simulink model "QCar2_Manual_Drive"  (R2023a)
settings: Solver=ode2  StartTime=0.0  StopTime=inf  FixedStep=1/100  RelTol=1e-3  EnableMultiTasking=on
undefined symbols (not defined in the file): HIL, Host, qc_get_step_size
libraries: quarc_library x15, simulink x13
settings Model: SimulationMode=external  ExtModeTrigDuration=10000  Creator=mbohra  LastModifiedBy=ZinanCen
settings SolverCC: AlgebraicLoopSolver=TrustRegion  PositivePriorityOrder=on
settings DataIOCC: SaveOutput=off  SignalLogging=off  DSMLogging=off  SaveTime=off  ReturnWorkspaceOutputs=off
settings DebuggingCC: UnconnectedInputMsg=warning  UnconnectedOutputMsg=warning  UnconnectedLineMsg=warning  ArithmeticOperatorsInVariantConditions=warning
settings ModelReferenceCC: EnableRefExpFcnMdlSchedulingChecks=on
settings SFSimCC: CustomCodeUndefinedFunction=UseInterfaceOnly
settings RTWCC: Toolchain=QUARC win64 | nmake (64-bit Windows)  BuildConfiguration=Faster Runs

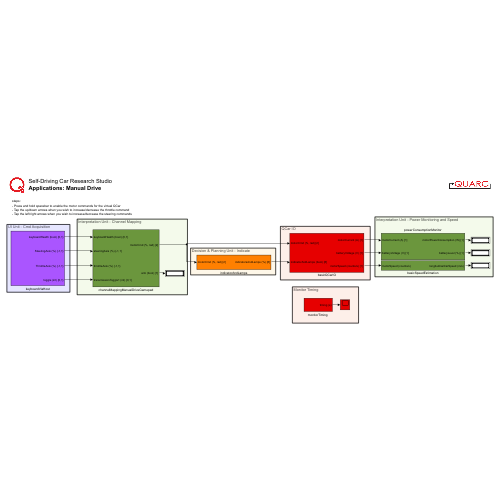
[thumbnail: Simulink's stored preview of the top-level diagram]
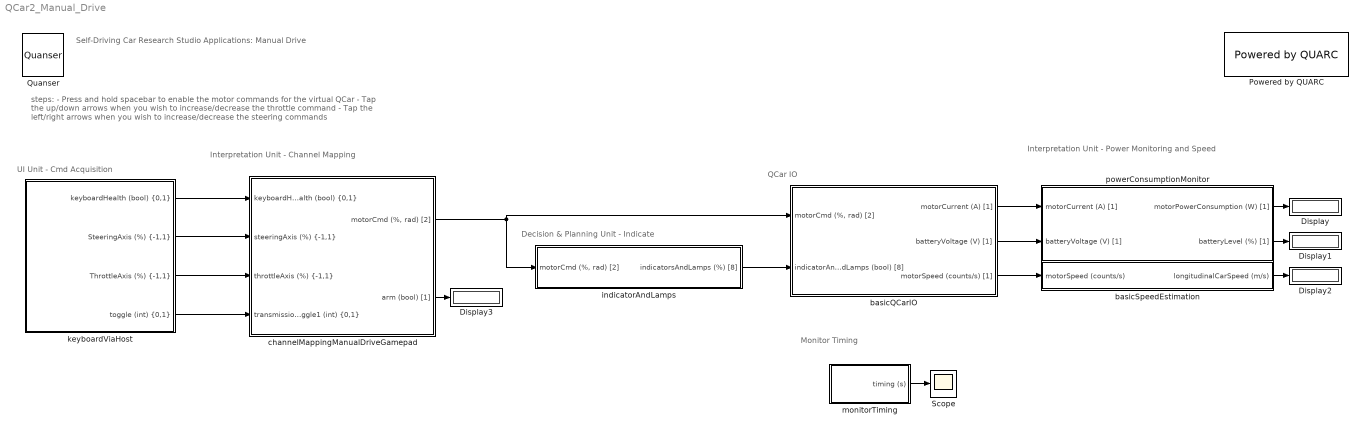
== system QCar2_Manual_Drive ==
  note: steps:
      | - Press and hold spacebar to enable the motor commands for the virtual QCar
      | - Tap the up/down arrows when you wish to increase/decrease the throttle command
      | - Tap the left/right arrows when you wish to increase/decrease the steering commands
  note: Monitor Timing
  note: Decision & Planning Unit - Indicate
  note: Interpretation Unit - Channel Mapping
  note: Interpretation Unit - Power Monitoring and Speed
  note: QCar IO
  note: UI Unit - Cmd Acquisition
  note: Self-Driving Car Research Studio
      | Applications: Manual Drive
  Display{,1..3} (4 alike) : Display
      Display settings: Decimation=0.5/qc_get_step_size
      Display1 settings: Decimation=0.5/qc_get_step_size
      Display2 settings: Decimation=0.5/qc_get_step_size
      Display3 settings: Decimation=0.1/qc_get_step_size
  Powered by QUARC : quarc_library/Logos/Powered by QUARC
  Quanser : quarc_library/Logos/Quanser
  Scope : Scope
  basicQCarIO : Subsystem
  basicSpeedEstimation : Subsystem
  channelMappingManualDriveGamepad : Subsystem
  indicatorAndLamps : Subsystem
  keyboardViaHost : Subsystem
  "monitorTiming " : Subsystem
  powerConsumptionMonitor : Subsystem
  wires:
  indicatorAndLamps/1(indicatorsAndLamps (%) [8]) -> basicQCarIO/2(indicatorAndLamps (bool) [8])
  keyboardViaHost/1("keyboardHealth (bool) {0,1}") -> channelMappingManualDriveGamepad/1("keyboardHealth (bool) {0,1}")
  channelMappingManualDriveGamepad/2(arm (bool) [1]) -> Display3/1
  basicQCarIO/3(motorSpeed (counts/s) [1]) -> basicSpeedEstimation/1(motorSpeed (counts/s))
  basicQCarIO/1(motorCurrent (A) [1]) -> powerConsumptionMonitor/1(motorCurrent (A) [1])
  basicQCarIO/2(batteryVoltage (V) [1]) -> powerConsumptionMonitor/2(batteryVoltage (V) [1])
  basicSpeedEstimation/1(longitudinalCarSpeed (m/s)) -> Display2/1
  powerConsumptionMonitor/2(batteryLevel (%) [1]) -> Display1/1
  powerConsumptionMonitor/1(motorPowerConsumption (W) [1]) -> Display/1
  "monitorTiming "/1(timing (s)) -> Scope/1
  channelMappingManualDriveGamepad/1("motorCmd (%, rad) [2]") -> basicQCarIO/1("motorCmd (%, rad) [2]"), indicatorAndLamps/1("motorCmd (%, rad) [2]")
  keyboardViaHost/3("ThrottleAxis (%) {-1,1}") -> channelMappingManualDriveGamepad/3("throttleAxis (%) {-1,1}")
  keyboardViaHost/2("SteeringAxis (%) {-1,1}") -> channelMappingManualDriveGamepad/2("steeringAxis (%) {-1,1}")
  keyboardViaHost/4("toggle (int) {0,1}") -> channelMappingManualDriveGamepad/4("transmissionToggle1 (int) {0,1}")

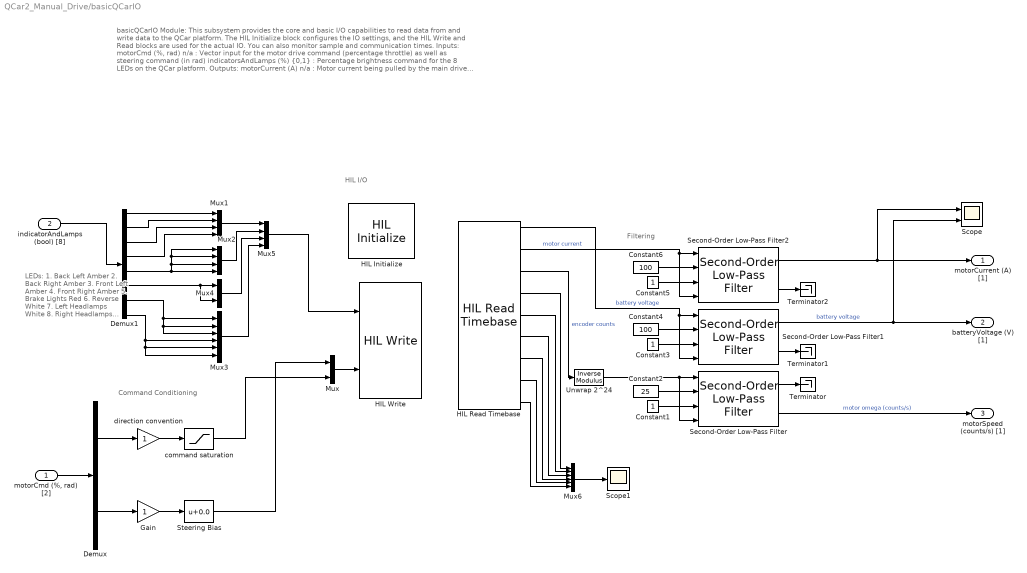
== system QCar2_Manual_Drive/basicQCarIO ==
  note: Filtering
  note: basicQCarIO Module:
      |
      | This subsystem provides the core and basic I/O capabilities to read data from and write data to the QCar platform. The HIL Initialize block configures the IO settings, and the HIL Write and Read blocks are used for the actual IO. You can also monitor sample and communication times.
      |
      | Inputs:
      | motorCmd (%, rad) n/a : Vector input for the motor drive command (percentage throttle) as well as steering command (in rad)
      | indicatorsAndLamps (%) {0,1} : Percentage brightness command for the 8 LEDs on the QCar platform.
      |
      | Outputs:
      | motorCurrent (A) n/a : Motor current being pulled by the main drive motor
      | batteryVoltage (V) {0, 12.6} : Current battery voltage reading
      | motorSpeed (counts/s) n/a : Drive motor speed measured using an encoder (do not confuse with wheel speed as this measurement is at the drive shaft)
  note: HIL I/O
  note: Command Conditioning
  note: LEDs:
      | 1. Back Left Amber
      | 2. Back Right Amber
      | 3. Front Left Amber
      | 4. Front Right Amber
      | 5. Brake Lights Red
      | 6. Reverse White
      | 7. Left Headlamps White
      | 8. Right Headlamps White
  "motorCmd (%, rad) [2]" : Inport
  indicatorAndLamps (bool) [8] : Inport  Port=2
  Constant1 : Constant
  Constant2 : Constant  Value=25
  Constant3 : Constant
  Constant4 : Constant  Value=100
  Constant5 : Constant
  Constant6 : Constant  Value=100
  Demux : Demux  Outputs=2
  Demux1 : Demux  Outputs=8
  Gain : Gain
  HIL Initialize : quarc_library/Data Acquisition/Generic/Configuration/HIL Initialize  object_name=HIL-1  board_type=qcar2  board_number=0@tcpip://localhost:18960  board_options=gyro_fs=250;gyro_rate=500;gyro_bw=125;gyro_ord=3;accel_fs=16;accel_rate=1000;accel_bw=250;accel_ord=3;temp_bw=4000;enc0_dir=0;enc1_dir=0;enc2_dir=0;steer_bias=0.05;  exclusive=off  active=on  hardware_clocks=[]  clock_modes=[]  initial_clock_frequencies=[]  set_clock_params_at_start=off  set_clock_params_at_switch_in=off  set_clock_frequencies_at_start=off  set_clock_frequencies_at_switch_in=off  analog_input_channels=[0:4]  analog_input_configurations=[]  analog_input_maximums=[3.3]  analog_input_minimums=[0]  set_analog_input_params_at_start=off  set_analog_input_params_at_switch_in=off  analog_output_channels=[]  analog_output_maximums=[]  analog_output_minimums=[]  initial_analog_outputs=[]  final_analog_outputs=[]  watchdog_analog_outputs=[]  set_analog_output_params_at_start=off  set_analog_output_params_at_switch_in=off  set_analog_outputs_at_start=off  set_analog_outputs_at_switch_in=off  set_analog_outputs_at_terminate=off  set_analog_outputs_at_switch_out=off  set_analog_outputs_on_watchdog=off  digital_input_channels=[0:14]  digital_output_channels=[11:26]  digital_output_configuration=[]  initial_digital_outputs=[0]  final_digital_outputs=[0]  watchdog_digital_outputs=[0]  set_digital_output_params_at_start=off  set_digital_output_params_at_switch_in=off  set_digital_outputs_at_start=on  set_digital_outputs_at_switch_in=off  set_digital_outputs_at_terminate=on  set_digital_outputs_at_switch_out=off  set_digital_outputs_on_watchdog=off  encoder_channels=[0:2]  quadrature=[4]  encoder_filter_frequency=100e6/1  initial_encoder_counts=[0]  set_encoder_params_at_start=on  set_encoder_params_at_switch_in=off  set_encoder_counts_at_start=on  set_encoder_counts_at_switch_in=off  pwm_channels=[0:1]  pwm_modes=[0]  pwm_frequency=180e6/4096  pwm_configuration=[0]  pwm_alignment=[0]  pwm_polarity=[1]  pwm_leading_deadband=[]  pwm_trailing_deadband=[]  initial_pwm_outputs=[0]  final_pwm_outputs=[0]  watchdog_pwm_outputs=[0]  set_pwm_params_at_start=on  set_pwm_params_at_switch_in=off  set_pwm_outputs_at_start=on  set_pwm_outputs_at_switch_in=off  set_pwm_outputs_at_terminate=on  set_pwm_outputs_at_switch_out=off  set_pwm_outputs_on_watchdog=off  other_output_channels=[1000 11000]  initial_other_outputs=[0]  final_other_outputs=[0]  watchdog_other_outputs=[0]  set_other_outputs_at_start=on  set_other_outputs_at_switch_in=off  set_other_outputs_at_terminate=on  set_other_outputs_at_switch_out=off  set_other_outputs_on_watchdog=off
  HIL Read Timebase : quarc_library/Data Acquisition/Generic/Timebases/HIL Read Timebase  object_name=HIL-1  clock=0  analog_channels=[2 4]  encoder_channels=[0]  digital_channels=[]  other_channels=[3000:3002 4000:4002]  active=on  vector_output=off  data_type_mode=Inherit via back propagation  encoder_data_type=double  digital_data_type=boolean  overflow_mode=Synchronize (for simulated cards only)  samples_in_buffer=max(ceil(1/qc_get_step_size), 1)*0+1
  HIL Write : quarc_library/Data Acquisition/Generic/Immediate I//O/HIL Write  object_name=HIL-1  analog_channels=[]  pwm_channels=[]  digital_channels=[17:18 25:26 11:16 19:24]  other_channels=[1000 11000]  sample_time=qc_get_step_size  active=on  vector_input=on
  Mux : Mux  Inputs=2
  Mux1 : Mux
  Mux2 : Mux
  Mux3 : Mux  Inputs=6
  Mux4 : Mux  Inputs=2
  Mux5 : Mux
  Mux6 : Mux  Inputs=6
  Scope : Scope  NumInputPorts=2
  Scope1 : Scope
  Second-Order Low-Pass Filter : quarc_library/Continuous/Second-Order Low-Pass Filter  params_source=External (input ports)  input_width=1  input_zeta=1  input_init=0
  Second-Order Low-Pass Filter1 : quarc_library/Continuous/Second-Order Low-Pass Filter  params_source=External (input ports)  input_width=1  input_zeta=1  input_init=0
  Second-Order Low-Pass Filter2 : quarc_library/Continuous/Second-Order Low-Pass Filter  params_source=External (input ports)  input_width=1  input_zeta=1  input_init=0
  Steering Bias : Bias  Bias=0.0  SaturateOnIntegerOverflow=off
  Terminator : Terminator
  Terminator1 : Terminator
  Terminator2 : Terminator
  Unwrap 2^24 : quarc_library/Discontinuities/Inverse Modulus  modulus=16777215  output_derivative=off  output_revolutions=off  max_x=Inf  min_x=-Inf
  command saturation : Saturate  UpperLimit=0.20  LowerLimit=-0.20
  direction convention : Gain
  motorCurrent (A) [1] : Outport  VectorParamsAs1DForOutWhenUnconnected=off
  batteryVoltage (V) [1] : Outport  Port=2  VectorParamsAs1DForOutWhenUnconnected=off
  motorSpeed (counts/s) [1] : Outport  Port=3  VectorParamsAs1DForOutWhenUnconnected=off
  wires:
  Second-Order Low-Pass Filter2/1 -> Scope/1, motorCurrent (A) [1]/1
  Constant2/1 -> Second-Order Low-Pass Filter/2
  Unwrap 2^24/1 -> Second-Order Low-Pass Filter/1, Second-Order Low-Pass Filter/4
  Second-Order Low-Pass Filter/1 -> Terminator/1
  Constant3/1 -> Second-Order Low-Pass Filter1/3
  Second-Order Low-Pass Filter1/1 -> Scope/2, batteryVoltage (V) [1]/1  "battery voltage"
  Constant5/1 -> Second-Order Low-Pass Filter2/3
  Second-Order Low-Pass Filter1/2 -> Terminator1/1
  HIL Read Timebase/1 -> Second-Order Low-Pass Filter1/4, Second-Order Low-Pass Filter1/1  "battery voltage"
  Constant6/1 -> Second-Order Low-Pass Filter2/2
  Second-Order Low-Pass Filter/2 -> motorSpeed (counts/s) [1]/1  "motor omega (counts/s)"
  Second-Order Low-Pass Filter2/2 -> Terminator2/1
  Constant4/1 -> Second-Order Low-Pass Filter1/2
  Constant1/1 -> Second-Order Low-Pass Filter/3
  HIL Read Timebase/3 -> Unwrap 2^24/1  "encoder counts"
  HIL Read Timebase/2 -> Second-Order Low-Pass Filter2/1, Second-Order Low-Pass Filter2/4  "motor current"
  Mux5/1 -> HIL Write/1
  "motorCmd (%, rad) [2]"/1 -> Demux/1
  Mux3/1 -> Mux5/4
  Demux1/4 -> Mux1/4
  Demux1/3 -> Mux1/3
  Demux1/6 -> Mux4/2, Mux4/1
  Steering Bias/1 -> Mux/1
  Demux1/8 -> Mux3/5, Mux3/6, Mux3/4
  Mux1/1 -> Mux5/1
  Demux1/7 -> Mux3/2, Mux3/3, Mux3/1
  Demux/1 -> direction convention/1
  Demux1/5 -> Mux2/4, Mux2/3, Mux2/2, Mux2/1
  Mux2/1 -> Mux5/2
  Mux/1 -> HIL Write/2
  indicatorAndLamps (bool) [8]/1 -> Demux1/1
  Demux/2 -> Gain/1
  Mux4/1 -> Mux5/3
  command saturation/1 -> Mux/2
  Demux1/2 -> Mux1/2
  direction convention/1 -> command saturation/1
  Gain/1 -> Steering Bias/1
  Demux1/1 -> Mux1/1
  Mux6/1 -> Scope1/1
  HIL Read Timebase/9 -> Mux6/6
  HIL Read Timebase/7 -> Mux6/4
  HIL Read Timebase/5 -> Mux6/2
  HIL Read Timebase/8 -> Mux6/5
  HIL Read Timebase/6 -> Mux6/3
  HIL Read Timebase/4 -> Mux6/1

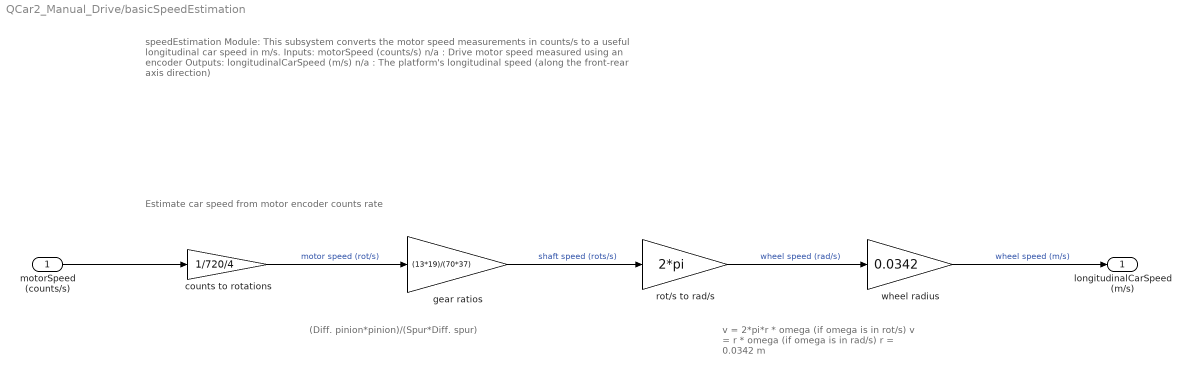
== system QCar2_Manual_Drive/basicSpeedEstimation ==
  note: speedEstimation Module:
      |
      | This subsystem converts the motor speed measurements in counts/s to a useful longitudinal car speed in m/s.
      |
      | Inputs:
      | motorSpeed (counts/s) n/a : Drive motor speed measured using an encoder
      |
      | Outputs:
      | longitudinalCarSpeed (m/s) n/a : The platform's longitudinal speed (along the front-rear axis direction)
  note: (Diff. pinion*pinion)/(Spur*Diff. spur)
  note: v = 2*pi*r * omega (if omega is in rot/s)
      | v = r * omega (if omega is in rad/s)
      | r = 0.0342 m
  note: Estimate car speed from motor encoder counts rate
  motorSpeed (counts/s) : Inport
  counts to rotations : Gain  Gain=1/720/4
  gear ratios : Gain  Gain=(13*19)/(70*37)
  rot/s to rad/s : Gain  Gain=2*pi
  wheel radius : Gain  Gain=0.0342
  longitudinalCarSpeed (m/s) : Outport  VectorParamsAs1DForOutWhenUnconnected=off
  wires:
  gear ratios/1 -> rot/s to rad/s/1  "shaft speed (rots/s)"
  wheel radius/1 -> longitudinalCarSpeed (m/s)/1  "wheel speed (m/s)"
  counts to rotations/1 -> gear ratios/1  "motor speed (rot/s)"
  rot/s to rad/s/1 -> wheel radius/1  "wheel speed (rad/s)"
  motorSpeed (counts/s)/1 -> counts to rotations/1

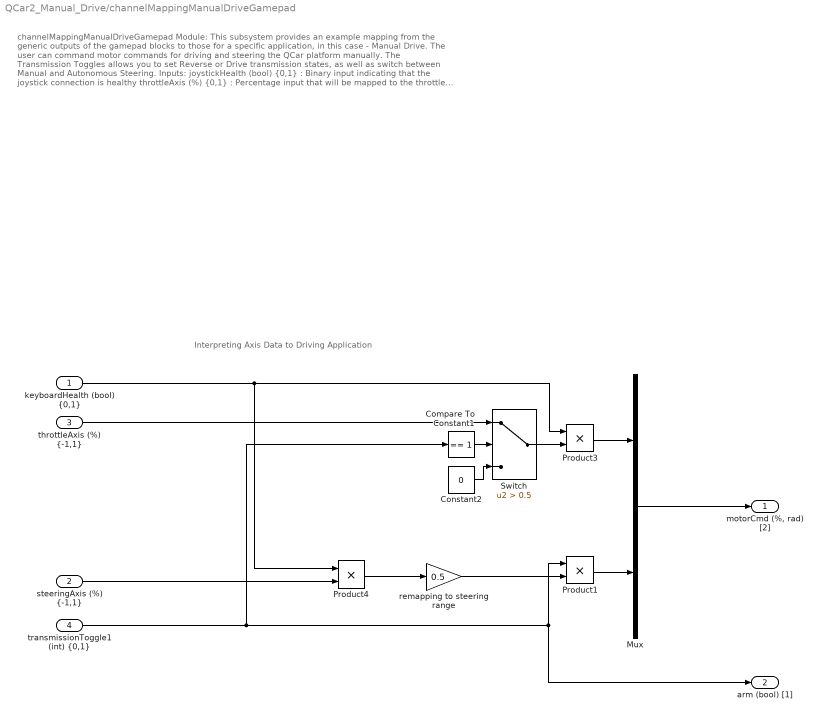
== system QCar2_Manual_Drive/channelMappingManualDriveGamepad ==
  note: channelMappingManualDriveGamepad Module:
      |
      | This subsystem provides an example mapping from the generic outputs of the gamepad blocks to those for a specific application, in this case - Manual Drive. The user can command motor commands for driving and steering the QCar platform manually. The Transmission Toggles allows you to set Reverse or Drive transmission states, as well as switch between Manual and Autonomous Steering.
      |
      | Inputs:
      | joystickHealth (bool) {0,1} : Binary input indicating that the joystick connection is healthy
      | throttleAxis (%) {0,1} : Percentage input that will be mapped to the throttle command
      | steeringAxis (%) {-1,1} : Signed percentage input that will be mapped to steering
      | transmissionToggle1 (int) {0,1} : 2-state input that will decide the Park/Engage State
      | transmissionToggle2 (int) {0, 1} : 2-state input that will decide the Reverse/Drive State
      |
      | Outputs:
      | motorCmd (%, rad) n/a : Vector output for the motor drive command (percentage throttle) as well as steering command (in rad)
      | arm (bool) {0,1} : Binary output indicating status (armed or disarmed)
      |
      | Usage:
      | 1. When the Transmission Toggle 1 input
      | a. reads 1, the Arm output will be high (1), which is the Armed state.
      | b. reads 0, the Arm output will be low (0), which is the Disarmed state.
      | 2. In addition, the Transmission Toggle 2 input
      | a. reading 0 is the Drive state, and the Motor Cmd for the throttle will range from 0 to 100%, spinning the wheels forwards.
      | b. reading 1 is the Reverse state, and the Motor Cmd for the throttle will range from 0 to -100%, spinning the wheels backwards.
  note: Interpreting Axis Data to Driving Application
  "keyboardHealth (bool) {0,1}" : Inport
  "steeringAxis (%) {-1,1}" : Inport  Port=2
  "throttleAxis (%) {-1,1}" : Inport  Port=3
  "transmissionToggle1 (int) {0,1}" : Inport  Port=4
  " remapping to steering range " : Gain  Gain=0.5
  Compare To Constant1 : simulink/Logic and Bit Operations/Compare To Constant  relop===  const=1  OutDataTypeStr=boolean
  Constant2 : Constant  Value=0
  Mux : Mux  Inputs=2
  Product1 : Product
  Product3 : Product
  Product4 : Product
  Switch : Switch  Criteria=u2 > Threshold  Threshold=0.5  SaturateOnIntegerOverflow=off  InputSameDT=off
  "motorCmd (%, rad) [2]" : Outport  VectorParamsAs1DForOutWhenUnconnected=off
  arm (bool) [1] : Outport  Port=2  VectorParamsAs1DForOutWhenUnconnected=off
  wires:
  Switch/1 -> Product3/2
  Product1/1 -> Mux/2
  Compare To Constant1/1 -> Switch/2
  "steeringAxis (%) {-1,1}"/1 -> Product4/2
  "keyboardHealth (bool) {0,1}"/1 -> Product4/1, Product3/1
  "transmissionToggle1 (int) {0,1}"/1 -> Compare To Constant1/1, Product1/1, arm (bool) [1]/1
  Product3/1 -> Mux/1
  " remapping to steering range "/1 -> Product1/2
  Product4/1 -> " remapping to steering range "/1
  Mux/1 -> "motorCmd (%, rad) [2]"/1
  "throttleAxis (%) {-1,1}"/1 -> Switch/1
  Constant2/1 -> Switch/3

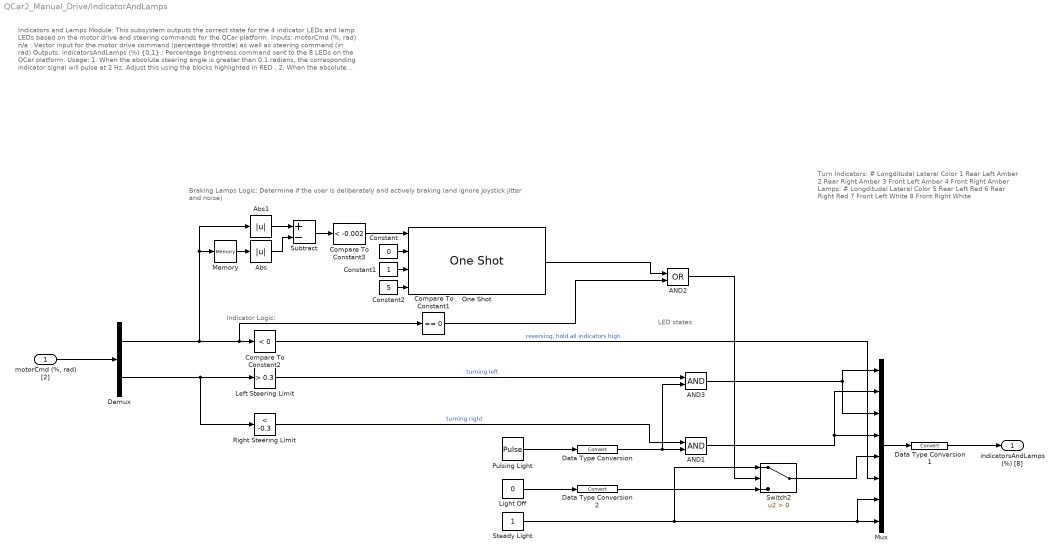
== system QCar2_Manual_Drive/indicatorAndLamps ==
  note: Indicators and Lamps Module:
      |
      | This subsystem outputs the correct state for the 4 indicator LEDs and lamp LEDs based on the motor drive and steering commands for the QCar platform.
      |
      | Inputs:
      | motorCmd (%, rad) n/a : Vector input for the motor drive command (percentage throttle) as well as steering command (in rad)
      |
      | Outputs:
      | indicatorsAndLamps (%) {0,1} : Percentage brightness command sent to the 8 LEDs on the QCar platform.
      |
      | Usage:
      | 1. When the absolute steering angle is greater than 0.1 radians, the corresponding indicator signal will pulse at 2 Hz. Adjust this using the blocks highlighted in RED .
      | 2. When the absolute motor drive command approaches 0, the brake lamps will receive 100% brightness command, and 0% brightness otherwise. Adjust this using the blocks highlighted in GREEN .
  note: Braking Lamps Logic:
      | Determine if the user is deliberately and actively braking (and ignore joystick jitter and noise)
  note: LED states
  note: Turn Indicators:
      | # Longditudal Lateral Color
      | 1 Rear Left Amber
      | 2 Rear Right Amber
      | 3 Front Left Amber
      | 4 Front Right Amber
      |
      | Lamps:
      | # Longditudal Lateral Color
      | 5 Rear Left Red
      | 6 Rear Right Red
      | 7 Front Left White
      | 8 Front Right White
  note: Indicator Logic:
  "motorCmd (%, rad) [2]" : Inport
  AND1 : Logic  IconShape=distinctive  AllPortsSameDT=off  OutDataTypeStr=boolean
  AND2 : Logic  Operator=OR  IconShape=distinctive  AllPortsSameDT=off  OutDataTypeStr=boolean
  AND3 : Logic  IconShape=distinctive  AllPortsSameDT=off  OutDataTypeStr=boolean
  Abs : Abs  SaturateOnIntegerOverflow=off
  Abs1 : Abs  SaturateOnIntegerOverflow=off
  Compare To Constant1 : simulink/Logic and Bit Operations/Compare To Constant  relop===  const=0  OutDataTypeStr=uint8
  Compare To Constant2 : simulink/Logic and Bit Operations/Compare To Constant  relop=<  const=0  OutDataTypeStr=boolean
  Compare To Constant3 : simulink/Logic and Bit Operations/Compare To Constant  relop=<  const=-0.002  OutDataTypeStr=boolean
  Constant : Constant  Value=0
  Constant1 : Constant
  Constant2 : Constant  Value=5
  Data Type Conversion : DataTypeConversion  SaturateOnIntegerOverflow=off  RndMeth=Floor
  Data Type Conversion1 : DataTypeConversion  SaturateOnIntegerOverflow=off  RndMeth=Floor
  Data Type Conversion2 : DataTypeConversion  SaturateOnIntegerOverflow=off  RndMeth=Floor
  Demux : Demux  Outputs=2
  Left Steering Limit : simulink/Logic and Bit Operations/Compare To Constant  relop=>  const=0.3  OutDataTypeStr=boolean
  Light Off : Constant  Value=0  OutDataTypeStr=boolean
  Memory : Memory
  Mux : Mux  Inputs=8
  One Shot : quarc_library/Discontinuities/One Shot  trigger_type=Falling edge  redun_pulse=Ignore extraneous pulse  width_source=External input port  pulse_width=100
      settings: SourceProductName=QUARC Targets
  Pulsing Light : DiscretePulseGenerator  Period=0.5/qc_get_step_size  PulseWidth=0.5/2/qc_get_step_size  SampleTime=qc_get_step_size
  Right Steering Limit : simulink/Logic and Bit Operations/Compare To Constant  relop=<  const=-0.3  OutDataTypeStr=boolean
  Steady Light : Constant  OutDataTypeStr=boolean
  Subtract : Sum  Inputs=+-
  Switch2 : Switch  Criteria=u2 > Threshold  SaturateOnIntegerOverflow=off  InputSameDT=off
  indicatorsAndLamps (%) [8] : Outport  VectorParamsAs1DForOutWhenUnconnected=off
  wires:
  Data Type Conversion2/1 -> Switch2/3
  Demux/2 -> Right Steering Limit/1, Left Steering Limit/1
  Light Off/1 -> Data Type Conversion2/1
  One Shot/1 -> AND2/1
  Steady Light/1 -> Mux/7, Mux/8, Switch2/1
  Compare To Constant3/1 -> One Shot/1
  Constant2/1 -> One Shot/4
  Right Steering Limit/1 -> AND1/1  "turning right"
  Mux/1 -> Data Type Conversion1/1
  Constant/1 -> One Shot/2
  Pulsing Light/1 -> Data Type Conversion/1
  Abs/1 -> Subtract/2
  Memory/1 -> Abs/1
  Abs1/1 -> Subtract/1
  Data Type Conversion/1 -> AND3/2, AND1/2
  Data Type Conversion1/1 -> indicatorsAndLamps (%) [8]/1
  Left Steering Limit/1 -> AND3/1  "turning left"
  Switch2/1 -> Mux/5
  Constant1/1 -> One Shot/3
  Demux/1 -> Compare To Constant1/1, Compare To Constant2/1, Memory/1, Abs1/1
  AND3/1 -> Mux/1, Mux/3
  "motorCmd (%, rad) [2]"/1 -> Demux/1
  Subtract/1 -> Compare To Constant3/1
  AND1/1 -> Mux/2, Mux/4
  Compare To Constant2/1 -> Mux/6  "reversing, hold all indicators high"
  Compare To Constant1/1 -> AND2/2
  AND2/1 -> Switch2/2

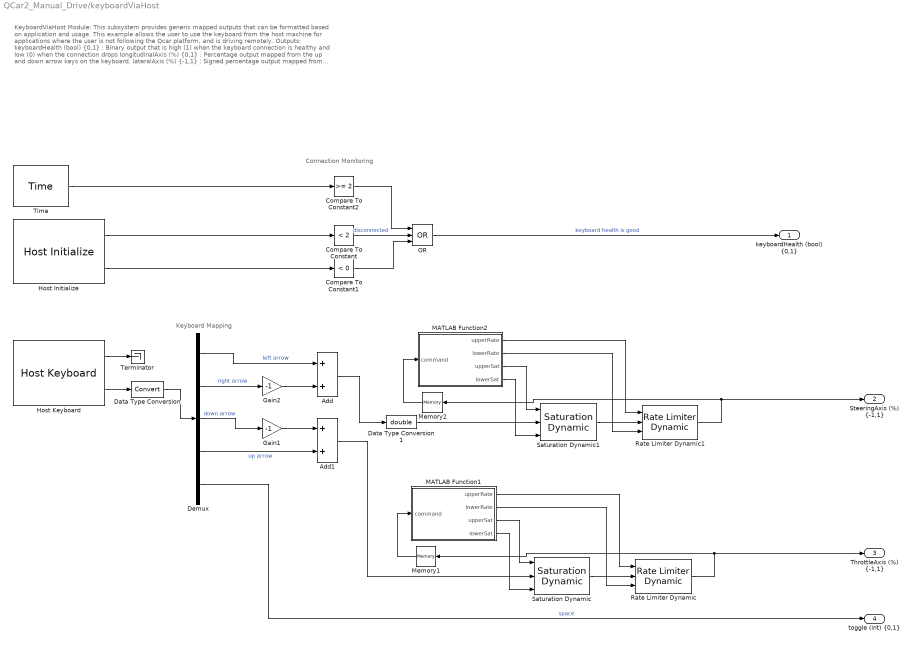
== system QCar2_Manual_Drive/keyboardViaHost ==
  note: Connection Monitoring
  note: KeyboardViaHost Module:
      |
      | This subsystem provides generic mapped outputs that can be formatted based on application and usage. This example allows the user to use the keyboard from the host machine for applications where the user is not following the Qcar platform, and is driving remotely.
      |
      | Outputs:
      | keyboardHealth (bool) {0,1} : Binary output that is high (1) when the keyboard connection is healthy and low (0) when the connection drops
      | longitudinalAxis (%) {0,1} : Percentage output mapped from the up and down arrow keys on the keyboard.
      | lateralAxis (%) {-1,1} : Signed percentage output mapped from the left and right arrow keys on the keyboard.
      | toggle (int) {0,1} : binary "arm" signal mapped to Space Bar.
      |
      | Note: Holding the arrow keys longer will increase/decrease the value further. Releasing the key will maintain values.
  note: Keyboard Mapping
  Add : Sum
  Add1 : Sum
  Compare To Constant : simulink/Logic and Bit Operations/Compare To Constant  relop=<  const=2  OutDataTypeStr=boolean
  Compare To Constant1 : simulink/Logic and Bit Operations/Compare To Constant  relop=<  const=0  OutDataTypeStr=boolean
  Compare To Constant2 : simulink/Logic and Bit Operations/Compare To Constant  relop=>=  const=2  OutDataTypeStr=boolean
  Data Type Conversion : DataTypeConversion  SaturateOnIntegerOverflow=off  RndMeth=Floor
  Data Type Conversion1 : DataTypeConversion  OutDataTypeStr=double  SaturateOnIntegerOverflow=off  RndMeth=Floor
  Demux : Demux  Outputs=5
  Gain1 : Gain  Gain=-1
  Gain2 : Gain  Gain=-1
  Host Initialize : quarc_library/Devices/Peripherals/Host/Host Initialize  object_name=Host-2  uri_source=Use external mode communications  uri=tcpip://localhost:18001  send_buffer_size=1000  receive_buffer_size=1000  thread_priority=0  run_client=on  use_window=off  window_position=[]  sample_time=qc_get_step_size  active=on
      settings: SourceProductName=QUARC Targets
  Host Keyboard : quarc_library/Devices/Peripherals/Host/Host Keyboard  object_name=Host-2  virtual_key="[37  39  40  38  32]"  sample_time=qc_get_step_size  enabled=on  debug_mode=off
      settings: SourceProductName=QUARC Targets
  MATLAB Function1 : MATLAB Function  TreatAsAtomicUnit=on
  MATLAB Function2 : MATLAB Function  TreatAsAtomicUnit=on
  Memory1 : Memory
  Memory2 : Memory
  OR : Logic  Operator=OR  Inputs=3  IconShape=distinctive  AllPortsSameDT=off  OutDataTypeStr=boolean
  Rate Limiter Dynamic : simulink/Discontinuities/Rate Limiter Dynamic
  Rate Limiter Dynamic1 : simulink/Discontinuities/Rate Limiter Dynamic
  Saturation Dynamic : simulink/Discontinuities/Saturation Dynamic  OutMin=[]  OutMax=[]  OutDataTypeStr=Inherit: Same as second input  OutDataType=fixdt(1, 16)  OutScaling=2^-10  DoSatur=off
  Saturation Dynamic1 : simulink/Discontinuities/Saturation Dynamic  OutMin=[]  OutMax=[]  OutDataTypeStr=Inherit: Same as second input  OutDataType=fixdt(1, 16)  OutScaling=2^-10  DoSatur=off
  Terminator : Terminator
  Time : quarc_library/Sources/Time/Time  time_source=Wall clock  sample_time=qc_get_step_size
  "keyboardHealth (bool) {0,1}" : Outport  VectorParamsAs1DForOutWhenUnconnected=off
  "SteeringAxis (%) {-1,1}" : Outport  Port=2  VectorParamsAs1DForOutWhenUnconnected=off
  "ThrottleAxis (%) {-1,1}" : Outport  Port=3  VectorParamsAs1DForOutWhenUnconnected=off
  "toggle (int) {0,1}" : Outport  Port=4  VectorParamsAs1DForOutWhenUnconnected=off
  wires:
  Host Initialize/1 -> Compare To Constant/1
  Demux/2 -> Gain2/1  "right arrow"
  Compare To Constant/1 -> OR/2  "disconnected"
  Demux/1 -> Add/1  "left arrow"
  Host Keyboard/2 -> Data Type Conversion/1
  Gain1/1 -> Add1/1
  OR/1 -> "keyboardHealth (bool) {0,1}"/1  "keyboard health is good"
  Demux/5 -> "toggle (int) {0,1}"/1  "space"
  Compare To Constant2/1 -> OR/1
  Time/1 -> Compare To Constant2/1
  Host Keyboard/1 -> Terminator/1
  Compare To Constant1/1 -> OR/3
  Data Type Conversion/1 -> Demux/1
  Host Initialize/2 -> Compare To Constant1/1
  Demux/3 -> Gain1/1  "down arrow"
  Demux/4 -> Add1/2  "up arrow"
  Gain2/1 -> Add/2
  Rate Limiter Dynamic/1 -> "ThrottleAxis (%) {-1,1}"/1, Memory1/1
  MATLAB Function1/4(lowerSat) -> Saturation Dynamic/3
  MATLAB Function1/3(upperSat) -> Saturation Dynamic/1
  MATLAB Function1/2(lowerRate) -> Rate Limiter Dynamic/3
  Saturation Dynamic/1 -> Rate Limiter Dynamic/2
  Add1/1 -> Saturation Dynamic/2
  MATLAB Function1/1(upperRate) -> Rate Limiter Dynamic/1
  Memory1/1 -> MATLAB Function1/1(command)
  Memory2/1 -> MATLAB Function2/1(command)
  MATLAB Function2/1(upperRate) -> Rate Limiter Dynamic1/1
  Add/1 -> Data Type Conversion1/1
  Saturation Dynamic1/1 -> Rate Limiter Dynamic1/2
  MATLAB Function2/2(lowerRate) -> Rate Limiter Dynamic1/3
  MATLAB Function2/3(upperSat) -> Saturation Dynamic1/1
  MATLAB Function2/4(lowerSat) -> Saturation Dynamic1/3
  Rate Limiter Dynamic1/1 -> "SteeringAxis (%) {-1,1}"/1, Memory2/1
  Data Type Conversion1/1 -> Saturation Dynamic1/2

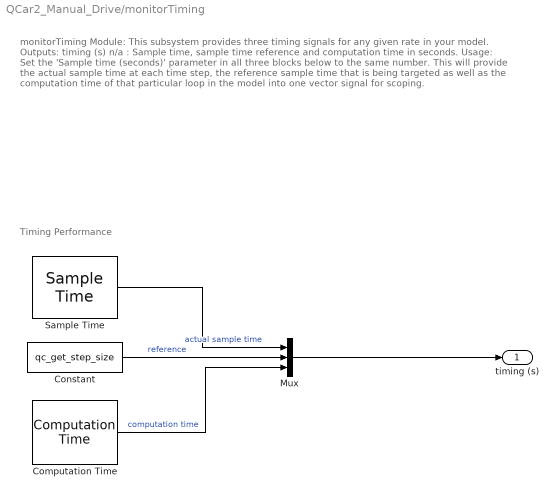
== system QCar2_Manual_Drive/monitorTiming  ==
  note: Timing Performance
  note: monitorTiming Module:
      |
      | This subsystem provides three timing signals for any given rate in your model.
      |
      | Outputs:
      | timing (s) n/a : Sample time, sample time reference and computation time in seconds.
      |
      | Usage:
      | Set the 'Sample time (seconds)' parameter in all three blocks below to the same number. This will provide the actual sample time at each time step, the reference sample time that is being targeted as well as the computation time of that particular loop in the model into one vector signal for scoping.
  Computation Time : quarc_library/Sources/Time/Computation Time  sample_time=qc_get_step_size  use_model=on  use_cpu_time=off
  Constant : Constant  Value=qc_get_step_size
  Mux : Mux  Inputs=3
  Sample Time : quarc_library/Sources/Time/Sample Time  Priority=-99  sample_time=qc_get_step_size
  timing (s) : Outport  VectorParamsAs1DForOutWhenUnconnected=off
  wires:
  Mux/1 -> timing (s)/1
  Computation Time/1 -> Mux/3  "computation time"
  Sample Time/1 -> Mux/1  "actual sample time"
  Constant/1 -> Mux/2  "reference"

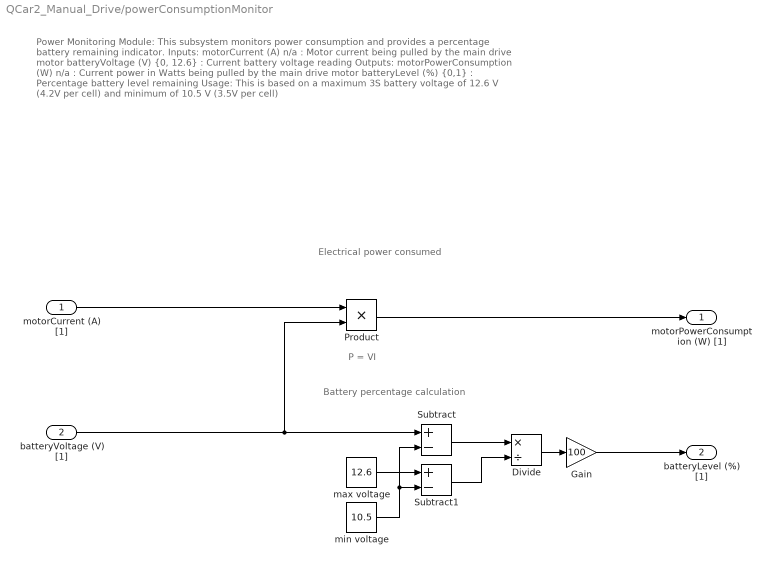
== system QCar2_Manual_Drive/powerConsumptionMonitor ==
  note: Battery percentage calculation
  note: P = VI
  note: Electrical
      | power
      | consumed
  note: Power Monitoring Module:
      |
      | This subsystem monitors power consumption and provides a percentage battery remaining indicator.
      |
      | Inputs:
      | motorCurrent (A) n/a : Motor current being pulled by the main drive motor
      | batteryVoltage (V) {0, 12.6} : Current battery voltage reading
      |
      | Outputs:
      | motorPowerConsumption (W) n/a : Current power in Watts being pulled by the main drive motor
      | batteryLevel (%) {0,1} : Percentage battery level remaining
      |
      | Usage:
      | This is based on a maximum 3S battery voltage of 12.6 V (4.2V per cell) and minimum of 10.5 V (3.5V per cell)
  motorCurrent (A) [1] : Inport
  batteryVoltage (V) [1] : Inport  Port=2
  Divide : Product  Inputs=*/
  Gain : Gain  Gain=100
  Product : Product
  Subtract : Sum  Inputs=+-
  Subtract1 : Sum  Inputs=+-
  max voltage : Constant  Value=12.6
  min voltage : Constant  Value=10.5
  motorPowerConsumption (W) [1] : Outport  VectorParamsAs1DForOutWhenUnconnected=off
  batteryLevel (%) [1] : Outport  Port=2  VectorParamsAs1DForOutWhenUnconnected=off
  wires:
  Divide/1 -> Gain/1
  Subtract1/1 -> Divide/2
  Gain/1 -> batteryLevel (%) [1]/1
  Product/1 -> motorPowerConsumption (W) [1]/1
  min voltage/1 -> Subtract/2, Subtract1/2
  motorCurrent (A) [1]/1 -> Product/1
  max voltage/1 -> Subtract1/1
  Subtract/1 -> Divide/1
  batteryVoltage (V) [1]/1 -> Subtract/1, Product/2

== matlab function QCar2_Manual_Drive/keyboardViaHost/MATLAB Function2 ==
  data: command input; upperRate output; lowerRate output; upperSat output; lowerSat output
function [upperRate, lowerRate, upperSat, lowerSat] = fcn(command)
% this function sets upper/lower saturation/rate limits for wheel speeds

% saturate the speeds the same way based on mode
upperSat    =  1;
lowerSat    = -1;
accel_limit = 22.50;

% saturate the accelerations (rate limit) based on speed commands
% to always allow faster braking
if command > 0
    upperRate =      accel_limit;
    lowerRate =  -10*accel_limit;
elseif command < 0 
    upperRate =   10*accel_limit;
    lowerRate =     -accel_limit;
else
    upperRate =      accel_limit;
    lowerRate =     -accel_limit;
end

== matlab function QCar2_Manual_Drive/keyboardViaHost/MATLAB Function1 ==
  data: command input; upperRate output; lowerRate output; upperSat output; lowerSat output
function [upperRate, lowerRate, upperSat, lowerSat] = fcn(command)
% this function sets upper/lower saturation/rate limits for wheel speeds

% saturate the speeds the same way based on mode
upperSat    =  1;
lowerSat    = -1;
accel_limit = 22.50;

% saturate the accelerations (rate limit) based on speed commands
% to always allow faster braking
if command > 0
    upperRate =      accel_limit;
    lowerRate =  -10*accel_limit;
elseif command < 0 
    upperRate =   10*accel_limit;
    lowerRate =     -accel_limit;
else
    upperRate =      accel_limit;
    lowerRate =     -accel_limit;
end
